simulink model "Motor"  (R2016b)
settings: Solver=VariableStepAuto  StartTime=0.0  StopTime=1  RelTol=1e-3
undefined symbols (not defined in the file or in its folder): dend, deng, dens, numd, numg, nums
settings Model: Creator=zeng  LastModifiedBy=zeng
settings SolverCC: InitialStep=1e-4

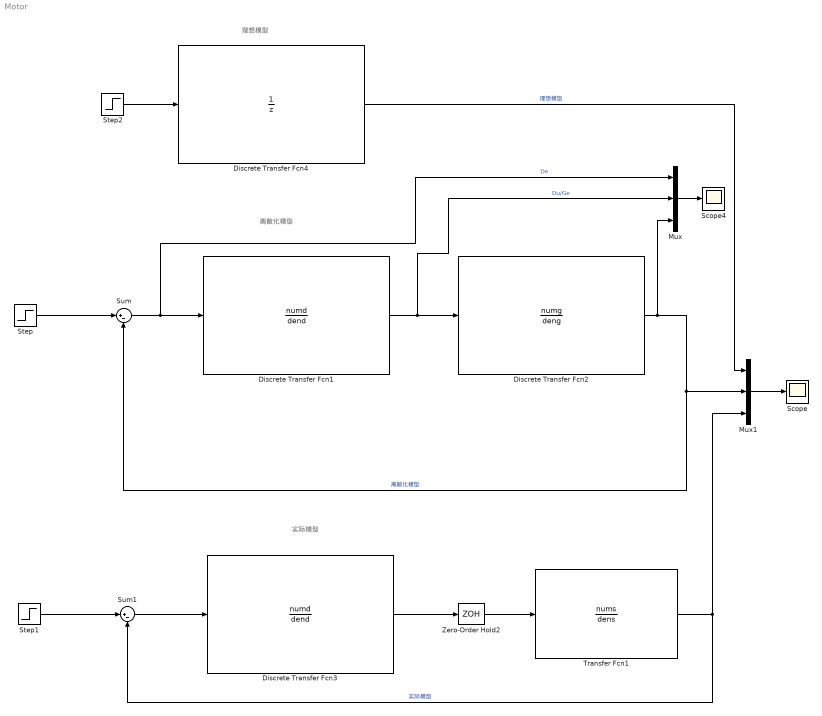
== system Motor ==
  note: 离散化模型
  note: 理想模型
  note: 实际模型
  Discrete Transfer Fcn1 : DiscreteTransferFcn  Numerator=numd  Denominator=dend  SampleTime=0.1
  Discrete Transfer Fcn2 : DiscreteTransferFcn  Numerator=numg  Denominator=deng  SampleTime=0.1
  Discrete Transfer Fcn3 : DiscreteTransferFcn  Numerator=numd  Denominator=dend  SampleTime=0.1
  Discrete Transfer Fcn4 : DiscreteTransferFcn  Numerator=1  Denominator=[1 0]  SampleTime=0.1
  Mux : Mux  Inputs=3
  Mux1 : Mux  Inputs=3
  Scope : Scope
  Scope4 : Scope
  Step : Step  Time=0.5  SampleTime=0
  Step1 : Step  Time=0.5  SampleTime=0
  Step2 : Step  Time=0.5  SampleTime=0
  Sum : Sum  Inputs=|+-
  Sum1 : Sum  Inputs=|+-
  Transfer Fcn1 : TransferFcn  Numerator=nums  Denominator=dens
  Zero-Order Hold2 : ZeroOrderHold  SampleTime=0.1
  wires:
  Step/1 -> Sum/1
  Sum/1 -> Mux/1, Discrete Transfer Fcn1/1  "De"
  Discrete Transfer Fcn1/1 -> Mux/2, Discrete Transfer Fcn2/1  "Du/Ge"
  Step1/1 -> Sum1/1
  Zero-Order Hold2/1 -> Transfer Fcn1/1
  Sum1/1 -> Discrete Transfer Fcn3/1
  Discrete Transfer Fcn3/1 -> Zero-Order Hold2/1
  Transfer Fcn1/1 -> Mux1/3, Sum1/2  "实际模型"
  Discrete Transfer Fcn2/1 -> Mux1/2, Sum/2, Mux/3  "离散化模型"
  Step2/1 -> Discrete Transfer Fcn4/1
  Mux/1 -> Scope4/1
  Mux1/1 -> Scope/1
  Discrete Transfer Fcn4/1 -> Mux1/1  "理想模型"
